simulink model "DroneSimulinkModel"  (R2025b)
settings: Solver=VariableStepAuto  StartTime=0.0  StopTime=10.0  RelTol=1e-3
InitFcn:
  | kf=1e-5;
  | m=0.5;
  | Irod=(2/3)*10^-4;
  | l=0.1;
libraries: simulink x4
settings Model: Creator=Alek  LastModifiedBy=Alek

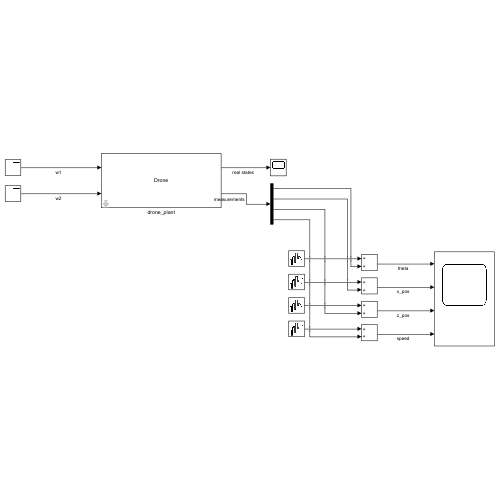
[thumbnail: Simulink's stored preview of the top-level diagram]
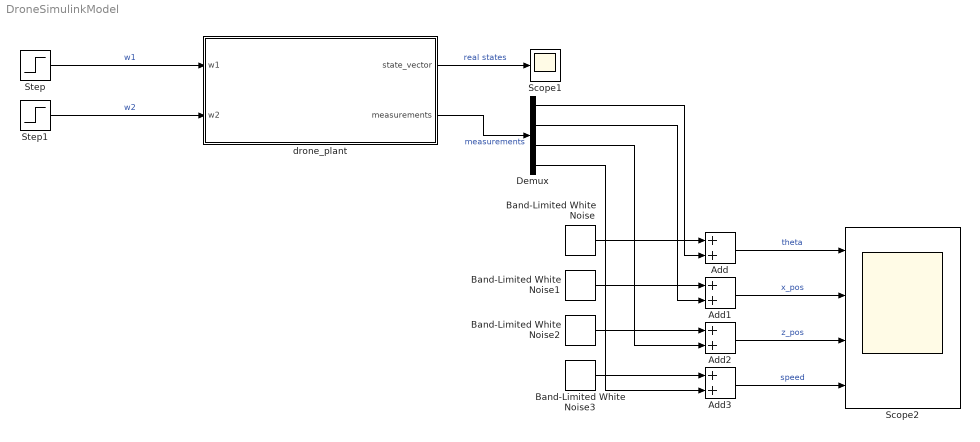
== system DroneSimulinkModel ==
  Add{,1..3} (4 alike) : Sum
  Band-Limited White Noise : simulink/Sources/Band-Limited White Noise  Cov=0.1  Ts=0.1  seed=[23341]
  Band-Limited White Noise1 : simulink/Sources/Band-Limited White Noise  Cov=3  Ts=0.1  seed=[23341]
  Band-Limited White Noise2 : simulink/Sources/Band-Limited White Noise  Cov=5  Ts=0.1  seed=[23341]
  Band-Limited White Noise3 : simulink/Sources/Band-Limited White Noise  Cov=2  Ts=0.1  seed=[23341]
  Demux : Demux
  Scope1 : Scope
      settings: ActiveDisplayYMinimum=-1  ActiveDisplayYMaximum=1
  Scope2 : Scope  NumInputPorts=4
      settings: ActiveDisplayYMinimum=-70.277121841634283  ActiveDisplayYMaximum=582.11436111126466  DataLoggingVariableName=ScopeData2
  Step : Step  Time=5  Before=490  After=495  SampleTime=0
  Step1 : Step  Time=5  Before=490  After=495  SampleTime=0
  drone_plant : Subsystem  mask{kf=1e-5, m=0.5, l=1e-2, Irod=6.6666e-5}
      mask prompts: kf "Thrust Coefficient"; m "Mass"; l "Arm length"; Irod "Rod Moment Of Intertia"
      mask Display: disp('Drone');
  wires:
  drone_plant/2(measurements) -> Demux/1  "measurements"
  drone_plant/1(state_vector) -> Scope1/1  "real states"
  Step1/1 -> drone_plant/2(w2)  "w2"
  Step/1 -> drone_plant/1(w1)  "w1"
  Demux/1 -> Add/2
  Demux/2 -> Add1/2
  Demux/3 -> Add2/2
  Demux/4 -> Add3/2
  Band-Limited White Noise/1 -> Add/1
  Band-Limited White Noise1/1 -> Add1/1
  Band-Limited White Noise2/1 -> Add2/1
  Band-Limited White Noise3/1 -> Add3/1
  Add/1 -> Scope2/1  "theta"
  Add1/1 -> Scope2/2  "x_pos"
  Add2/1 -> Scope2/3  "z_pos"
  Add3/1 -> Scope2/4  "speed"

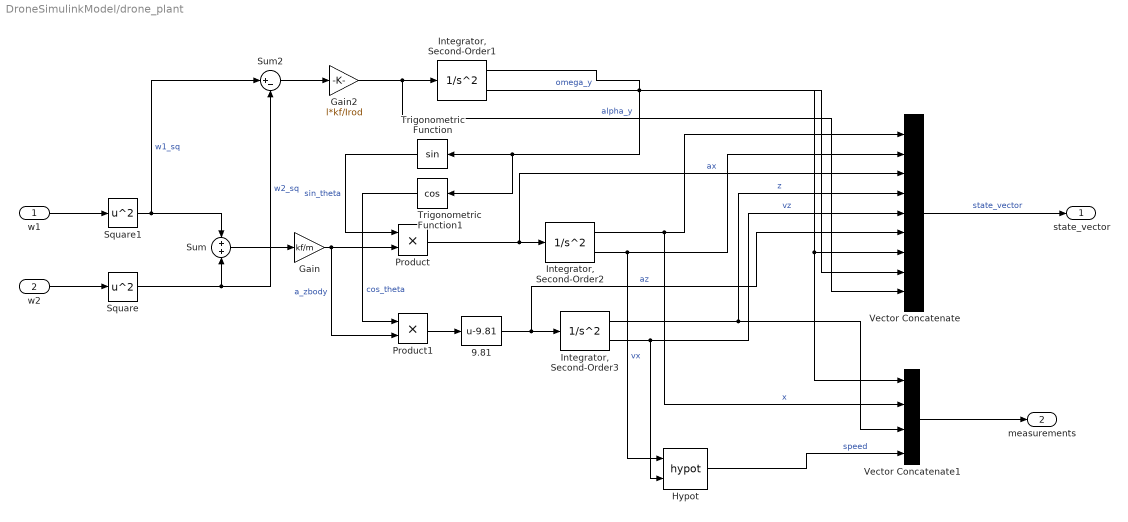
== system DroneSimulinkModel/drone_plant ==
  w1 : Inport
  w2 : Inport  Port=2
  9.81 : Bias  Bias=-9.81  SaturateOnIntegerOverflow=off
  Gain : Gain  Gain=kf/m
  Gain2 : Gain  Gain=l*kf/Irod
  Hypot : Math  Operator=hypot
  "Integrator, Second-Order1" : SecondOrderIntegrator
  "Integrator, Second-Order2" : SecondOrderIntegrator  ICX=0
  "Integrator, Second-Order3" : SecondOrderIntegrator  ICX=500  LimitX=on  LowerLimitX=0
  Product : Product
  Product1 : Product
  Square : Math  Operator=square
  Square1 : Math  Operator=square
  Sum : Sum  Inputs=+|+
  Sum2 : Sum  Inputs=|+-
  Trigonometric Function : Trigonometry
  Trigonometric Function1 : Trigonometry  Operator=cos
  Vector Concatenate : Concatenate  NumInputs=9
  Vector Concatenate1 : Concatenate  NumInputs=4
  state_vector : Outport
  measurements : Outport  Port=2
  wires:
  Square1/1 -> Sum2/1, Sum/1  "w1_sq"
  9.81/1 -> Vector Concatenate/6, "Integrator, Second-Order3"/1  "az"
  "Integrator, Second-Order1"/1 -> Vector Concatenate1/1, Vector Concatenate/7, Trigonometric Function1/1, Trigonometric Function/1
  "Integrator, Second-Order2"/2 -> Vector Concatenate/2, Hypot/1  "vx"
  Sum/1 -> Gain/1
  Trigonometric Function/1 -> Product/1  "sin_theta"
  Product1/1 -> 9.81/1
  Gain2/1 -> Vector Concatenate/9, "Integrator, Second-Order1"/1  "alpha_y"
  Product/1 -> Vector Concatenate/3, "Integrator, Second-Order2"/1  "ax"
  Square/1 -> Sum2/2, Sum/2  "w2_sq"
  Vector Concatenate1/1 -> measurements/1
  Gain/1 -> Product1/2, Product/2  "a_zbody"
  "Integrator, Second-Order3"/1 -> Vector Concatenate1/3, Vector Concatenate/4  "z"
  Trigonometric Function1/1 -> Product1/1  "cos_theta"
  "Integrator, Second-Order3"/2 -> Hypot/2, Vector Concatenate/5  "vz"
  Hypot/1 -> Vector Concatenate1/4  "speed"
  Sum2/1 -> Gain2/1
  w1/1 -> Square1/1
  Vector Concatenate/1 -> state_vector/1  "state_vector"
  w2/1 -> Square/1
  "Integrator, Second-Order2"/1 -> Vector Concatenate1/2, Vector Concatenate/1  "x"
  "Integrator, Second-Order1"/2 -> Vector Concatenate/8  "omega_y"
